simulink model "kalman"  (R2024a)
settings: Solver=VariableStepAuto  StartTime=0.0  StopTime=10.0  RelTol=1e-7
values from neighbouring files (symbols this model uses):
  A = [4, -2, 0, 6; -2, 4, -6, 0; 0, -6, 4, 2; 6, 0, 2, 4]    [main.m]
  C = [1, -1, 1, 1; 1, 3, -1, 3]    [main.m]
  L = -P * C' / R    [TAU.m]    (also in main.m = TAU.FindObserverKalman(A, C, QL, RL))
  vare = 0.5    [main.m]
  varf = 1    [main.m]
  x0 = [1; 1; 1; 1]    [main.m]
settings Model: Creator=alexivanov  LastModifiedBy=alexivanov

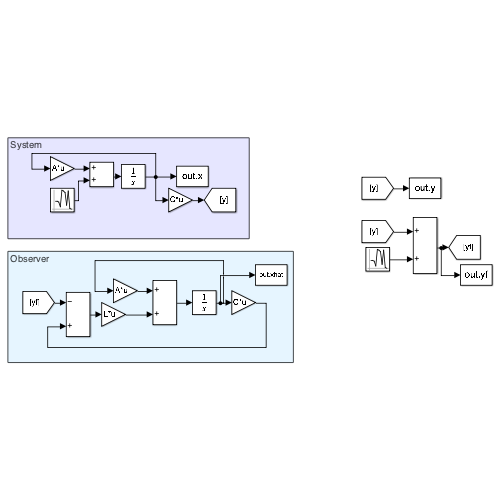
[thumbnail: Simulink's stored preview of the top-level diagram]
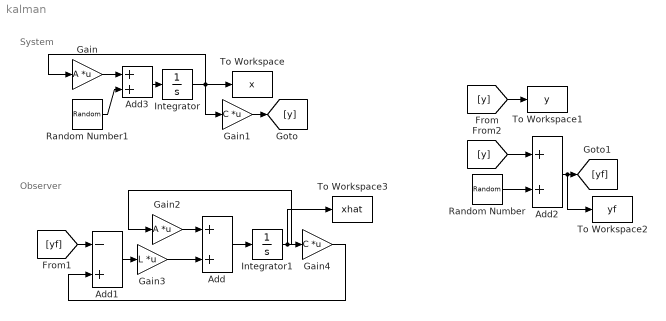
== system kalman ==
  note: Observer
  note: System
  Add : Sum
  Add1 : Sum  Inputs=-+
  Add2 : Sum
  Add3 : Sum
  Gain : Gain  Gain=A  Multiplication=Matrix(K*u)
  Gain1 : Gain  Gain=C  Multiplication=Matrix(K*u)
  Gain2 : Gain  Gain=A  Multiplication=Matrix(K*u)
  Gain3 : Gain  Gain=L  Multiplication=Matrix(K*u)
  Gain4 : Gain  Gain=C  Multiplication=Matrix(K*u)
  Integrator : Integrator  InitialCondition=x0
  Integrator1 : Integrator
  Random Number : RandomNumber  Variance=vare  SampleTime=0.001
  Random Number1 : RandomNumber  Variance=varf  SampleTime=0.001
  To Workspace : ToWorkspace  VariableName=x  SampleTime=-1
  To Workspace1 : ToWorkspace  VariableName=y  SampleTime=-1
  To Workspace2 : ToWorkspace  VariableName=yf  SampleTime=-1
  To Workspace3 : ToWorkspace  VariableName=xhat  SampleTime=-1
  wires:
  Gain/1 -> Add3/1
  Add2/1 -> To Workspace2/1, [yf]
  Integrator1/1 -> To Workspace3/1, Gain4/1, Gain2/1
  Gain3/1 -> Add/2
  Add3/1 -> Integrator/1
  Gain1/1 -> [y]
  [yf] -> Add1/1
  Random Number/1 -> Add2/2
  Gain4/1 -> Add1/2
  Add/1 -> Integrator1/1
  Integrator/1 -> Gain1/1, Gain/1, To Workspace/1
  Gain2/1 -> Add/1
  Random Number1/1 -> Add3/2
  Add1/1 -> Gain3/1
  [y] -> To Workspace1/1
  [y] -> Add2/1
